simulink model "Test_Memory_Blocks"  (Simulink 8.1)
settings: Solver=ode45  StartTime=0.0  StopTime=5  RelTol=1e-3
libraries: Computer_Library x3, simulink_extras x3
settings Model: Creator=N  LastModifiedBy=uzivatel
settings DataIOCC: LimitDataPoints=off  SignalLoggingSaveFormat=Dataset
settings OptimizationCC: ExpressionDepthLimit=128
settings DebuggingCC: UnderspecifiedInitializationDetection=Simplified  MergeDetectMultiDrivingBlocksExec=error  SolverPrmCheckMsg=none  FcnCallInpInsideContextMsg=EnableAllAsError  FrameProcessingCompatibilityMsg=error  StateNameClashWarn=none
settings HardwareCC: ProdBitPerPointer=64  ProdLargestAtomicFloat=Float  ProdIntDivRoundTo=Zero  ProdEndianess=LittleEndian  ProdHWDeviceType=Intel->x86-64 (Windows64)
settings ModelReferenceCC: PropagateSignalLabelsOutOfModel=on
settings GRTTargetCC: CodeReplacementLibrary=None  CombineOutputUpdateFcns=on  CPPClassGenCompliant=on  GRTInterface=off

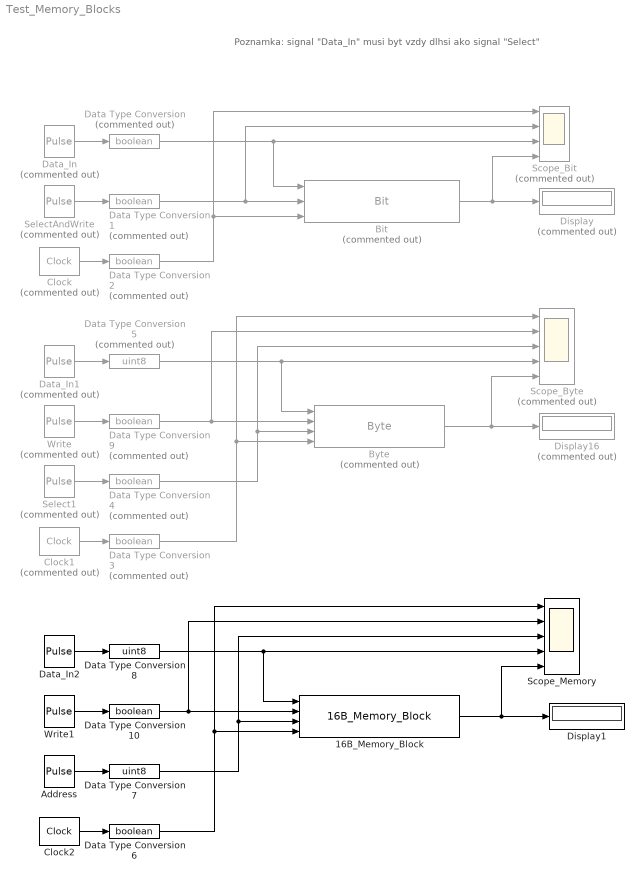
== system Test_Memory_Blocks ==
  note: Poznamka: signal "Data_In" musi byt vzdy dlhsi ako signal "Select"
  16B_Memory_Block : Computer_Library/Memory_Blocks/16B_Memory_Block
  Address : DiscretePulseGenerator  PulseType=Time based  Amplitude=10  PulseWidth=10  PhaseDelay=0.35
  Bit : Computer_Library/Memory_Blocks/Bit  Commented=on
  Byte : Computer_Library/Memory_Blocks/Byte  Commented=on
  Clock : simulink_extras/Flip Flops/Clock  Commented=on  period=1
  Clock1 : simulink_extras/Flip Flops/Clock  Commented=on  period=1
  Clock2 : simulink_extras/Flip Flops/Clock  period=1
  Data Type Conversion{,1..4,9} (6 alike) : DataTypeConversion  Commented=on  OutDataTypeStr=boolean
  Data Type Conversion10 : DataTypeConversion  OutDataTypeStr=boolean
  Data Type Conversion5 : DataTypeConversion  Commented=on  OutDataTypeStr=uint8
  Data Type Conversion6 : DataTypeConversion  OutDataTypeStr=boolean
  Data Type Conversion7 : DataTypeConversion  OutDataTypeStr=uint8
  Data Type Conversion8 : DataTypeConversion  OutDataTypeStr=uint8
  Data_In : DiscretePulseGenerator  Commented=on  PulseType=Time based  Period=5  PulseWidth=40  PhaseDelay=0.25
  Data_In1 : DiscretePulseGenerator  Commented=on  PulseType=Time based  Amplitude=255  Period=6  PulseWidth=40  PhaseDelay=0.25
  Data_In2 : DiscretePulseGenerator  PulseType=Time based  Amplitude=255  Period=6  PulseWidth=40  PhaseDelay=0.25
  Display : Display  Commented=on
  Display1 : Display
  Display16 : Display  Commented=on
  Scope_Bit : Scope  Commented=on  NumInputPorts=4
      settings: YMin=0~0~0~0  YMax=1.5~1.5~1.5~1.5
  Scope_Byte : Scope  Commented=on  NumInputPorts=5
      settings: YMin=0~0~0~0~0  YMax=1.5~1.5~1.5~300~300
  Scope_Memory : Scope  NumInputPorts=5
      settings: YMin=0~0~0~0~0  YMax=1.5~1.5~20~300~300  SaveName=ScopeData2
  Select1 : DiscretePulseGenerator  Commented=on  PulseType=Time based  Period=3  PulseWidth=10  PhaseDelay=0.25
  SelectAndWrite : DiscretePulseGenerator  Commented=on  PulseType=Time based  Period=3  PulseWidth=10  PhaseDelay=0.25
  Write : DiscretePulseGenerator  Commented=on  PulseType=Time based  Period=6  PulseWidth=10  PhaseDelay=0.25
  Write1 : DiscretePulseGenerator  PulseType=Time based  Period=6  PulseWidth=10  PhaseDelay=0.25
  wires:
  Bit/1 -> Scope_Bit/4, Display/1
  Data Type Conversion/1 -> Scope_Bit/3, Bit/1
  Data Type Conversion1/1 -> Scope_Bit/2, Bit/2
  Data Type Conversion4/1 -> Scope_Byte/3, Byte/3
  Byte/1 -> Scope_Byte/5, Display16/1
  Data Type Conversion5/1 -> Byte/1, Scope_Byte/4
  Data_In/1 -> Data Type Conversion/1
  SelectAndWrite/1 -> Data Type Conversion1/1
  Data Type Conversion2/1 -> Scope_Bit/1, Bit/3
  Clock/1 -> Data Type Conversion2/1
  Clock1/1 -> Data Type Conversion3/1
  Select1/1 -> Data Type Conversion4/1
  Data Type Conversion3/1 -> Byte/4, Scope_Byte/1
  Data_In1/1 -> Data Type Conversion5/1
  Clock2/1 -> Data Type Conversion6/1
  Address/1 -> Data Type Conversion7/1
  Data_In2/1 -> Data Type Conversion8/1
  Data Type Conversion7/1 -> Scope_Memory/3, 16B_Memory_Block/3
  16B_Memory_Block/1 -> Scope_Memory/5, Display1/1
  Data Type Conversion8/1 -> 16B_Memory_Block/1, Scope_Memory/4
  Data Type Conversion6/1 -> 16B_Memory_Block/4, Scope_Memory/1
  Write/1 -> Data Type Conversion9/1
  Data Type Conversion9/1 -> Scope_Byte/2, Byte/2
  Write1/1 -> Data Type Conversion10/1
  Data Type Conversion10/1 -> Scope_Memory/2, 16B_Memory_Block/2
